simulink model "state_s"  (R2018b)
settings: Solver=VariableStepAuto  StartTime=0.0  StopTime=1000  RelTol=1e-3
values from neighbouring files (symbols this model uses):
  D = [-(cp*ro_p*fpn+K1+Kw)/cv_w , K1/cv_w ; K1/cv_p ,-(K1+Kp)/cv_p ]    [domek.m]
  E = [ cp*ro_p*fpn/cv_w, Kw/cv_w ; 0 , Kp/cv_p ]    [domek.m]
  Tzew = TzewN +dT    (= -17)    [domek.m]
  TzN = 80    [domek.m]
  War_Tp = T(2,1)    [domek.m]
  War_Twew = T(1,1)    [domek.m]
settings Model: Creator=stasz  LastModifiedBy=stasz

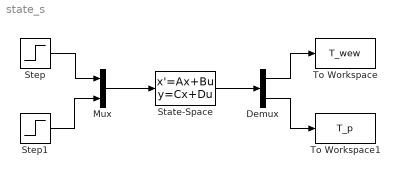
== system state_s ==
  Demux : Demux  Outputs=2
  Mux : Mux  Inputs=2
  State-Space : StateSpace  A=D  B=E  C=eye(2)  D=zeros(2)  InitialCondition=[War_Twew ; War_Tp]
  Step : Step  Before=TzN  After=TzN  SampleTime=0
  Step1 : Step  Before=Tzew  After=Tzew  SampleTime=0
  To Workspace : ToWorkspace  VariableName=T_wew  SaveFormat=Timeseries  SampleTime=-1
  To Workspace1 : ToWorkspace  VariableName=T_p  SaveFormat=Timeseries  SampleTime=-1
  wires:
  Step/1 -> Mux/1
  Step1/1 -> Mux/2
  Mux/1 -> State-Space/1
  State-Space/1 -> Demux/1
  Demux/2 -> To Workspace1/1
  Demux/1 -> To Workspace/1
